simulink model "resolved_acceleration_control_final"  (R2016a)
settings: Solver=ode45  StartTime=0.0  StopTime=25  FixedStep=0.001  RelTol=1e-3
InitFcn:
  | clear all;
  | Kpx = 10;
  | Kix = 25;
  | Kpy = 10;
  | Kiy = 25;
  | Kvphi = 3;
  | Kpphi = 2.25;
  | 
  | Kem = 0.0059;
  | Kti = 0.0059;
  | Vd = 5.4;
  | R = 1.71;
  | r = 0.072;
  | eta = 0.83;
  | N = 19;
  | 
  | Jw = 8.1e-4
undefined symbols (not defined in the file or in its folder): alpha1, alpha2, alpha3, l1, l2, l3
libraries: simulink x1
settings Model: Creator=Pichau  LastModifiedBy=Pichau

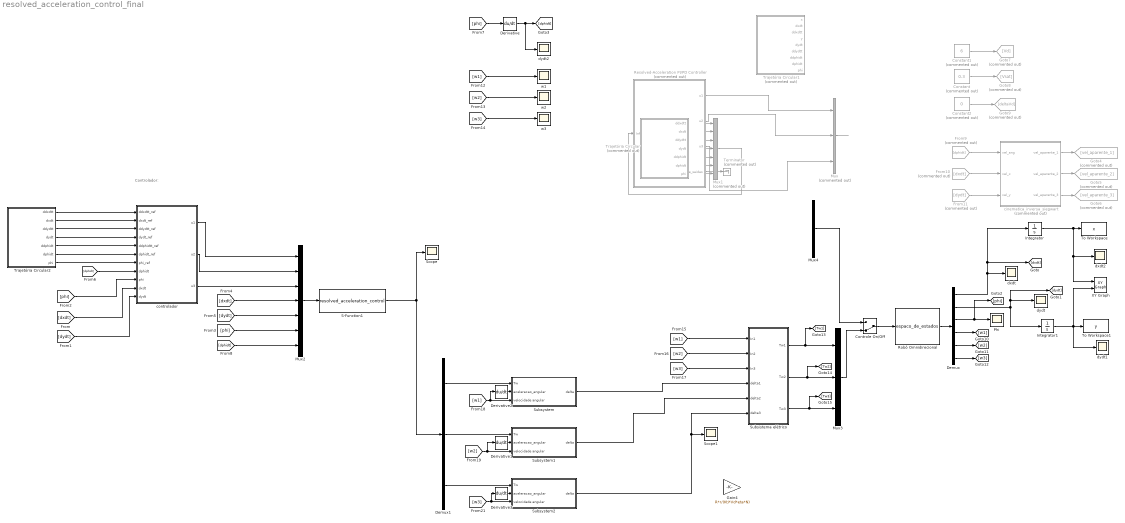
== system resolved_acceleration_control_final ==
  note: Controlador:
  Constant : Constant  Commented=on  Value=0.3
  Constant1 : Constant  Commented=on  Value=6
  Constant2 : Constant  Commented=on  Value=0
  Controle On/Off : ManualSwitch  CurrentSetting=0
  Demux : Demux  Outputs=6
  Demux1 : Demux  Outputs=3
  Derivative{,1..3} (4 alike) : Derivative
  From10 : From  Commented=on  GotoTag=dxdt
  From11 : From  Commented=on  GotoTag=dydt
  From9 : From  Commented=on  GotoTag=dphidt
  Gain4 : Gain  Gain=R*r/(Kti*Vd*eta*N)
  Goto4 : Goto  Commented=on  GotoTag=vel_aparente_1
  Goto5 : Goto  Commented=on  GotoTag=vel_aparente_2
  Goto6 : Goto  Commented=on  GotoTag=vel_aparente_3
  Goto7 : Goto  Commented=on  GotoTag=Vd
  Goto8 : Goto  Commented=on  GotoTag=Vsat
  Goto9 : Goto  Commented=on  GotoTag=deltaVd
  Integrator : Integrator  InitialCondition=0.3
  Integrator1 : Integrator
  Mux : Mux  Commented=on  Inputs=3
  Mux1 : Mux  Commented=on  Inputs=7
  Mux2 : Mux  Inputs=7
  Mux3 : Mux  Inputs=3
  Mux4 : Mux  Inputs=3
  Phi : Scope
  Resolved-Acceleration PI/PD Controller : Subsystem  Commented=on  mask{m=9.4, r=0.0245, L=11.25, J=11.25, Jw=0.02108, Kpx=10, Kix=25, Kpy=10, Kiy=25, Kvphi=3, Kpphi=2.25}
  Robô Omnidirecional : S-Function  FunctionName=espaco_de_estados  Parameters=r,m,Jw,J,L  SFunctionDeploymentMode=off  EnableBusSupport=off  mask{r=0.072, m=1.71, Jw=8.1e-4, J=2.125, L=0.09}
      mask prompts: r "r (m)"; m "m (Kg)"; Jw "Jw (Kg*m^2)"; J "J (Kg*m^2)"; L "L (m)"
      mask Display: image(imread('Robot_omnidirectional_drive.png'));
  S-Function1 : S-Function  FunctionName=resolved_acceleration_control  Parameters=r,L,m,J,Jw  SFunctionDeploymentMode=off  EnableBusSupport=off  mask{r=0.072, L=0.09, m=1.71, J=2.125, Jw=8.1e-4}
  Scope : Scope
  Scope1 : Scope
  Subsistema elétrico : Subsystem
  Subsystem : Subsystem
  Subsystem1 : Subsystem
  Subsystem2 : Subsystem
  Terminator : Terminator  Commented=on
  To Workspace : ToWorkspace  VariableName=x  SaveFormat=Timeseries  SampleTime=-1
  To Workspace1 : ToWorkspace  VariableName=y  SaveFormat=Timeseries  SampleTime=-1
  Trajetória Circular : Subsystem  Commented=on
  Trajetória Circular1 : Subsystem  Commented=on
  Trajetória Circular2 : Subsystem
  XY Graph : simulink/Sinks/XY Graph  xmin=-1  xmax=1  ymin=-1  ymax=1  st=-1
  cinematica_inversa_siegwart : Subsystem  Commented=on
  controlador : Subsystem
  dxdt : Scope
  dxdt2 : Scope
  dydt : Scope
  dydt1 : Scope
  dydt2 : Scope
  w1 : Scope
  w2 : Scope
  w3 : Scope
  wires:
  Mux/1 -> ?
  Robô Omnidirecional/1 -> Demux/1
  Resolved-Acceleration PI/PD Controller/4(vetor_de_saidas) -> Terminator/1
  Trajetória Circular/1(ddxdtt) -> Mux1/1
  Trajetória Circular/2(dxdt) -> Mux1/2
  Trajetória Circular/3(ddydtt) -> Mux1/3
  Trajetória Circular/4(dydt) -> Mux1/4
  Trajetória Circular/5(ddphidt) -> Mux1/5
  Trajetória Circular/6(dphidt) -> Mux1/6
  Trajetória Circular/7(phi) -> Mux1/7
  Mux1/1 -> Resolved-Acceleration PI/PD Controller/1(Informação da trajetória)
  Integrator1/1 -> XY Graph/2, To Workspace1/1, dydt1/1
  Integrator/1 -> XY Graph/1, dxdt2/1, To Workspace/1
  Trajetória Circular2/2(dxdt) -> controlador/2(dxdt_ref)
  Trajetória Circular2/6(dphidt) -> controlador/6(dphidt_ref)
  Trajetória Circular2/1(ddxdtt) -> controlador/1(ddxdtt_ref)
  Trajetória Circular2/4(dydt) -> controlador/4(dydt_ref)
  Trajetória Circular2/3(ddydtt) -> controlador/3(ddydtt_ref)
  Trajetória Circular2/7(phi) -> controlador/7(phi_ref)
  Trajetória Circular2/5(ddphidt) -> controlador/5(ddphidtt_ref)
  controlador/1(u1) -> Mux2/1
  controlador/2(u2) -> Mux2/2
  controlador/3(u3) -> Mux2/3
  [dxdt] -> controlador/10(dxdt)
  [dydt] -> controlador/11(dydt)
  [phi] -> controlador/9(phi)
  Resolved-Acceleration PI/PD Controller/1(u1) -> Mux/1
  Resolved-Acceleration PI/PD Controller/2(u2) -> Mux/2
  Resolved-Acceleration PI/PD Controller/3(u3) -> Mux/3
  Mux2/1 -> S-Function1/1
  [dphidt] -> controlador/8(dphidt)
  Derivative/1 -> dydt2/1, [dphidt]
  S-Function1/1 -> Scope/1, Demux1/1
  Mux3/1 -> Controle On/Off/2
  Controle On/Off/1 -> Robô Omnidirecional/1
  From9/1 -> cinematica_inversa_siegwart/1(vel_ang)
  From10/1 -> cinematica_inversa_siegwart/2(vel_x)
  From11/1 -> cinematica_inversa_siegwart/3(vel_y)
  cinematica_inversa_siegwart/1(vel_aparente_1) -> Goto4/1
  cinematica_inversa_siegwart/2(vel_aparente_2) -> Goto5/1
  cinematica_inversa_siegwart/3(vel_aparente_3) -> Goto6/1
  Constant1/1 -> Goto7/1
  Constant/1 -> Goto8/1
  Constant2/1 -> Goto9/1
  [w3] -> w3/1
  [w2] -> w2/1
  [w1] -> w1/1
  Demux/1 -> [dxdt], Integrator/1, dxdt/1
  Demux/2 -> Integrator1/1, [dydt], dydt/1
  Demux/3 -> Phi/1, [phi]
  [phi] -> Derivative/1
  [dxdt] -> Mux2/4
  [dydt] -> Mux2/5
  [phi] -> Mux2/6
  [dphidt] -> Mux2/7
  Demux/4 -> [w1]
  Demux/5 -> [w2]
  Demux/6 -> [w3]
  [w1] -> Subsistema elétrico/1(In1)
  [w2] -> Subsistema elétrico/2(In2)
  [w3] -> Subsistema elétrico/3(In3)
  Subsistema elétrico/3(Tw3) -> [Tw3], Mux3/3
  Subsistema elétrico/2(Tw2) -> [Tw2], Mux3/2
  Subsistema elétrico/1(Tw1) -> [Tw1], Mux3/1
  Mux4/1 -> Controle On/Off/1
  Demux1/1 -> Subsystem/1(Tw)
  Demux1/2 -> Subsystem1/1(Tw)
  Demux1/3 -> Subsystem2/1(Tw)
  Subsystem1/1(delta) -> Subsistema elétrico/5(delta2)
  Subsystem2/1(delta) -> Subsistema elétrico/6(delta3), Scope1/1
  Subsystem/1(delta) -> Subsistema elétrico/4(delta1)
  [w1] -> Derivative2/1, Subsystem/3(velocidade angular)
  [w2] -> Derivative1/1, Subsystem1/3(velocidade angular)
  [w3] -> Derivative3/1, Subsystem2/3(velocidade angular)
  Derivative1/1 -> Subsystem1/2(aceleracao_angular)
  Derivative2/1 -> Subsystem/2(aceleracao_angular)
  Derivative3/1 -> Subsystem2/2(aceleracao_angular)

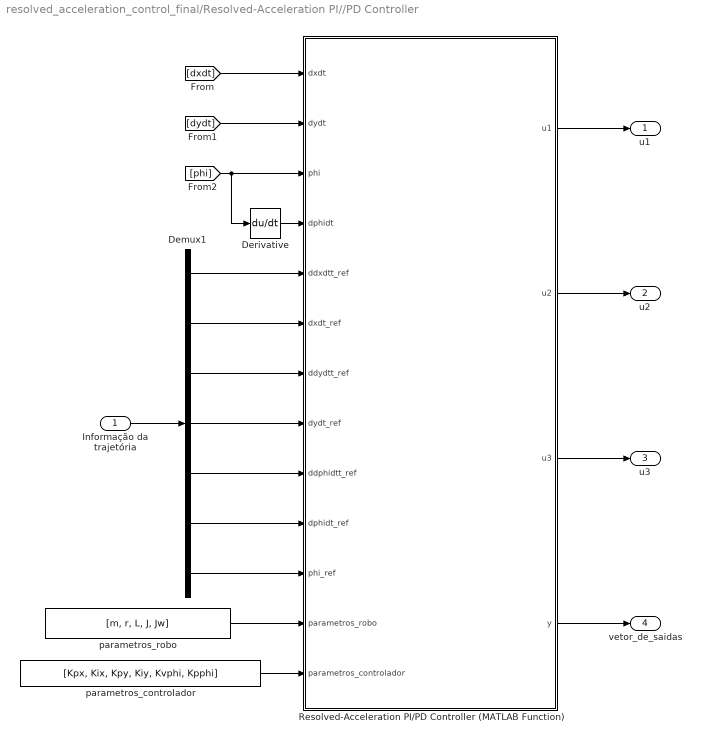
== system resolved_acceleration_control_final/Resolved-Acceleration PI//PD Controller ==
  Informação da trajetória : Inport
  Demux1 : Demux  Outputs=7
  Derivative : Derivative
  Resolved-Acceleration PI/PD Controller (MATLAB Function) : MATLAB Function  TreatAsAtomicUnit=on
  parametros_controlador : Constant  Value=[Kpx, Kix, Kpy, Kiy, Kvphi, Kpphi]
  parametros_robo : Constant  Value=[m, r, L, J, Jw]
  u1 : Outport
  u2 : Outport  Port=2
  u3 : Outport  Port=3
  vetor_de_saidas : Outport  Port=4
  wires:
  Resolved-Acceleration PI/PD Controller (MATLAB Function)/1(u1) -> u1/1
  parametros_controlador/1 -> Resolved-Acceleration PI/PD Controller (MATLAB Function)/13(parametros_controlador)
  [dxdt] -> Resolved-Acceleration PI/PD Controller (MATLAB Function)/1(dxdt)
  [phi] -> Derivative/1, Resolved-Acceleration PI/PD Controller (MATLAB Function)/3(phi)
  Resolved-Acceleration PI/PD Controller (MATLAB Function)/2(u2) -> u2/1
  Demux1/3 -> Resolved-Acceleration PI/PD Controller (MATLAB Function)/7(ddydtt_ref)
  Informação da trajetória/1 -> Demux1/1
  Resolved-Acceleration PI/PD Controller (MATLAB Function)/4(y) -> vetor_de_saidas/1
  parametros_robo/1 -> Resolved-Acceleration PI/PD Controller (MATLAB Function)/12(parametros_robo)
  Demux1/1 -> Resolved-Acceleration PI/PD Controller (MATLAB Function)/5(ddxdtt_ref)
  Demux1/2 -> Resolved-Acceleration PI/PD Controller (MATLAB Function)/6(dxdt_ref)
  Demux1/4 -> Resolved-Acceleration PI/PD Controller (MATLAB Function)/8(dydt_ref)
  Demux1/6 -> Resolved-Acceleration PI/PD Controller (MATLAB Function)/10(dphidt_ref)
  Derivative/1 -> Resolved-Acceleration PI/PD Controller (MATLAB Function)/4(dphidt)
  Resolved-Acceleration PI/PD Controller (MATLAB Function)/3(u3) -> u3/1
  Demux1/5 -> Resolved-Acceleration PI/PD Controller (MATLAB Function)/9(ddphidtt_ref)
  Demux1/7 -> Resolved-Acceleration PI/PD Controller (MATLAB Function)/11(phi_ref)
  [dydt] -> Resolved-Acceleration PI/PD Controller (MATLAB Function)/2(dydt)

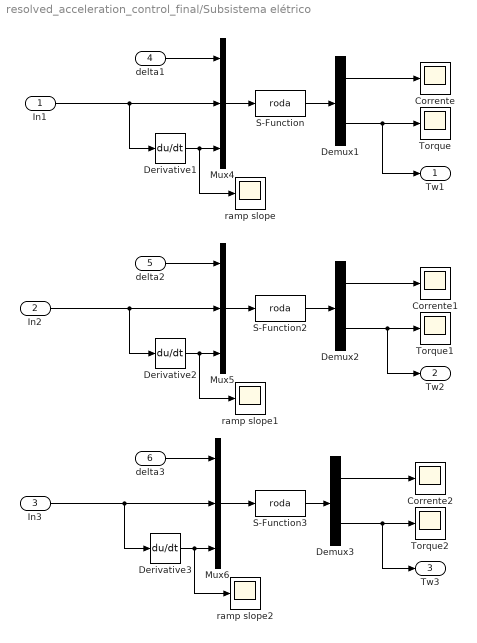
== system resolved_acceleration_control_final/Subsistema elétrico ==
  In1 : Inport
  In2 : Inport  Port=2
  In3 : Inport  Port=3
  delta1 : Inport  Port=4
  delta2 : Inport  Port=5
  delta3 : Inport  Port=6
  Corrente : Scope
  Corrente1 : Scope
  Corrente2 : Scope
  Demux1 : Demux  Outputs=2
  Demux2 : Demux  Outputs=2
  Demux3 : Demux  Outputs=2
  Derivative1 : Derivative
  Derivative2 : Derivative
  Derivative3 : Derivative
  Mux4 : Mux  Inputs=3
  Mux5 : Mux  Inputs=3
  Mux6 : Mux  Inputs=3
  S-Function : S-Function  FunctionName=roda  Parameters=Vd,Vsat,deltaVd,L,Kem,R,Kti,Jm,eta,N  SFunctionDeploymentMode=off  EnableBusSupport=off  mask{Vd=6, Vsat=0.3, deltaVd=0, L=0.00011, Kem=0.0059, R=1.71, Kti=0.0059, Jm=3.88e-7, eta=0.83, N=19}
  S-Function2 : S-Function  FunctionName=roda  Parameters=Vd,Vsat,deltaVd,L,Kem,R,Kti,Jm,eta,N  SFunctionDeploymentMode=off  EnableBusSupport=off  mask{Vd=6, Vsat=0.3, deltaVd=0, L=0.00011, Kem=0.0059, R=1.71, Kti=0.0059, Jm=3.88e-7, eta=0.83, N=19}
  S-Function3 : S-Function  FunctionName=roda  Parameters=Vd,Vsat,deltaVd,L,Kem,R,Kti,Jm,eta,N  SFunctionDeploymentMode=off  EnableBusSupport=off  mask{Vd=6, Vsat=0.3, deltaVd=0, L=0.00011, Kem=0.0059, R=1.71, Kti=0.0059, Jm=3.88e-7, eta=0.83, N=19}
  Torque : Scope
  Torque1 : Scope
  Torque2 : Scope
  ramp slope : Scope
  ramp slope1 : Scope
  ramp slope2 : Scope
  Tw1 : Outport
  Tw2 : Outport  Port=2
  Tw3 : Outport  Port=3
  wires:
  Demux3/1 -> Corrente2/1
  Mux6/1 -> S-Function3/1
  Derivative3/1 -> ramp slope2/1, Mux6/3
  Demux3/2 -> Tw3/1, Torque2/1
  In3/1 -> Mux6/2, Derivative3/1
  S-Function3/1 -> Demux3/1
  delta2/1 -> Mux5/1
  delta3/1 -> Mux6/1
  Mux5/1 -> S-Function2/1
  In2/1 -> Derivative2/1, Mux5/2
  S-Function2/1 -> Demux2/1
  Demux2/1 -> Corrente1/1
  Demux2/2 -> Tw2/1, Torque1/1
  Derivative2/1 -> Mux5/3, ramp slope1/1
  Derivative1/1 -> ramp slope/1, Mux4/3
  In1/1 -> Mux4/2, Derivative1/1
  Demux1/2 -> Tw1/1, Torque/1
  Mux4/1 -> S-Function/1
  S-Function/1 -> Demux1/1
  delta1/1 -> Mux4/1
  Demux1/1 -> Corrente/1

== system resolved_acceleration_control_final/Subsystem ==
  Tw : Inport
  aceleracao_angular : Inport  Port=2
  velocidade angular : Inport  Port=3
  Add : Sum  Inputs=+++
  Gain : Gain  Gain=R/(eta*N*Kti*Vd)
  Gain1 : Gain  Gain=Kem
  Gain2 : Gain  Gain=R*Jw/(eta*N^2*Kti*Vd)
  delta : Outport
  wires:
  aceleracao_angular/1 -> Gain2/1
  velocidade angular/1 -> Gain1/1
  Add/1 -> delta/1
  Tw/1 -> Gain/1
  Gain1/1 -> Add/3
  Gain/1 -> Add/1
  Gain2/1 -> Add/2

== system resolved_acceleration_control_final/Subsystem1 ==
  Tw : Inport
  aceleracao_angular : Inport  Port=2
  velocidade angular : Inport  Port=3
  Add : Sum  Inputs=+++
  Gain : Gain  Gain=R/(eta*N*Kti*Vd)
  Gain1 : Gain  Gain=Kem
  Gain2 : Gain  Gain=R*Jw/(eta*N^2*Kti*Vd)
  delta : Outport
  wires:
  Gain2/1 -> Add/2
  Gain/1 -> Add/1
  Gain1/1 -> Add/3
  Tw/1 -> Gain/1
  Add/1 -> delta/1
  velocidade angular/1 -> Gain1/1
  aceleracao_angular/1 -> Gain2/1

== system resolved_acceleration_control_final/Subsystem2 ==
  Tw : Inport
  aceleracao_angular : Inport  Port=2
  velocidade angular : Inport  Port=3
  Add : Sum  Inputs=+++
  Gain : Gain  Gain=R/(eta*N*Kti*Vd)
  Gain1 : Gain  Gain=Kem
  Gain2 : Gain  Gain=R*Jw/(eta*N^2*Kti*Vd)
  delta : Outport
  wires:
  aceleracao_angular/1 -> Gain2/1
  velocidade angular/1 -> Gain1/1
  Add/1 -> delta/1
  Tw/1 -> Gain/1
  Gain1/1 -> Add/3
  Gain/1 -> Add/1
  Gain2/1 -> Add/2

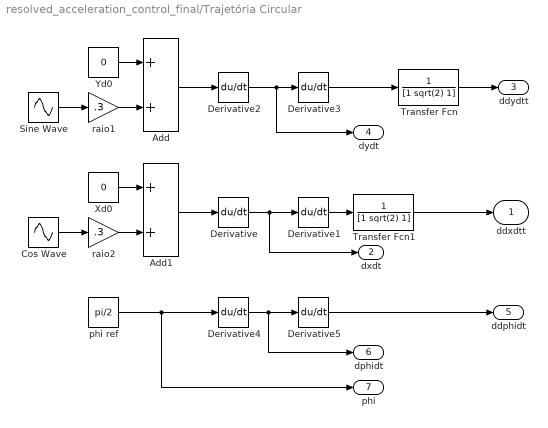
== system resolved_acceleration_control_final/Trajetória Circular ==
  Add : Sum
  Add1 : Sum
  Cos Wave : Sin  Frequency=0.3  Phase=pi/2  SampleTime=0
  Derivative{,1..5} (6 alike) : Derivative
  Sine Wave : Sin  Frequency=0.3  SampleTime=0
  Transfer Fcn : TransferFcn  Denominator=[1 sqrt(2) 1]
  Transfer Fcn1 : TransferFcn  Denominator=[1 sqrt(2) 1]
  Xd0 : Constant  Value=0
  Yd0 : Constant  Value=0
  phi ref : Constant  Value=pi/2
  raio1 : Gain  Gain=.3
  raio2 : Gain  Gain=.3
  ddxdtt : Outport
  dxdt : Outport  Port=2
  ddydtt : Outport  Port=3
  dydt : Outport  Port=4
  ddphidt : Outport  Port=5
  dphidt : Outport  Port=6
  phi : Outport  Port=7
  wires:
  Yd0/1 -> Add/1
  Xd0/1 -> Add1/1
  Cos Wave/1 -> raio2/1
  raio2/1 -> Add1/2
  Add1/1 -> Derivative/1
  Add/1 -> Derivative2/1
  raio1/1 -> Add/2
  Sine Wave/1 -> raio1/1
  Derivative/1 -> dxdt/1, Derivative1/1
  Derivative2/1 -> dydt/1, Derivative3/1
  Derivative3/1 -> Transfer Fcn/1
  Derivative1/1 -> Transfer Fcn1/1
  Derivative4/1 -> dphidt/1, Derivative5/1
  Derivative5/1 -> ddphidt/1
  phi ref/1 -> phi/1, Derivative4/1
  Transfer Fcn/1 -> ddydtt/1
  Transfer Fcn1/1 -> ddxdtt/1

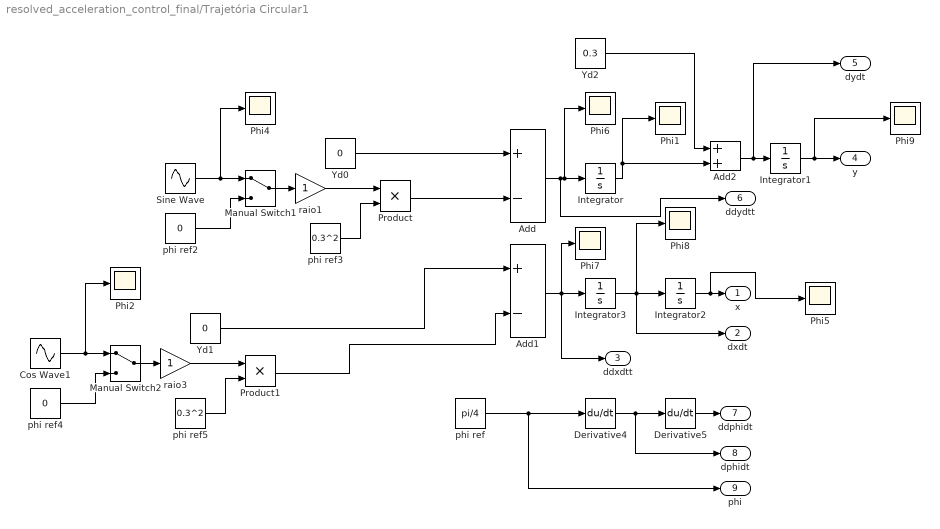
== system resolved_acceleration_control_final/Trajetória Circular1 ==
  Add : Sum  Inputs=+-
  Add1 : Sum  Inputs=+-
  Add2 : Sum
  Cos Wave1 : Sin  Frequency=0.3  Phase=pi/2  SampleTime=0
  Derivative4 : Derivative
  Derivative5 : Derivative
  Integrator : Integrator
  Integrator1 : Integrator
  Integrator2 : Integrator  InitialCondition=1
  Integrator3 : Integrator
  Manual Switch1 : ManualSwitch
  Manual Switch2 : ManualSwitch
  Phi{1..2,4..9} (8 alike) : Scope
  Product : Product
  Product1 : Product
  Sine Wave : Sin  Frequency=0.3  SampleTime=0
  Yd0 : Constant  Value=0
  Yd1 : Constant  Value=0
  Yd2 : Constant  Value=0.3
  phi ref : Constant  Value=pi/4
  phi ref2 : Constant  Value=0
  phi ref3 : Constant  Value=0.3^2
  phi ref4 : Constant  Value=0
  phi ref5 : Constant  Value=0.3^2
  raio1 : Gain
  raio3 : Gain
  x : Outport
  dxdt : Outport  Port=2
  ddxdtt : Outport  Port=3
  y : Outport  Port=4
  dydt : Outport  Port=5
  ddydtt : Outport  Port=6
  ddphidt : Outport  Port=7
  dphidt : Outport  Port=8
  phi : Outport  Port=9
  wires:
  phi ref/1 -> Derivative4/1, phi/1
  Derivative5/1 -> ddphidt/1
  Derivative4/1 -> Derivative5/1, dphidt/1
  Integrator/1 -> Phi1/1, Add2/2
  Integrator3/1 -> Phi8/1, Integrator2/1, dxdt/1
  Sine Wave/1 -> Phi4/1, Manual Switch1/1
  raio1/1 -> Product/1
  Add1/1 -> ddxdtt/1, Phi7/1, Integrator3/1
  Product1/1 -> Add1/2
  Yd1/1 -> Add1/1
  Yd0/1 -> Add/1
  Manual Switch1/1 -> raio1/1
  phi ref2/1 -> Manual Switch1/2
  Product/1 -> Add/2
  phi ref3/1 -> Product/2
  Cos Wave1/1 -> Phi2/1, Manual Switch2/1
  raio3/1 -> Product1/1
  Manual Switch2/1 -> raio3/1
  phi ref4/1 -> Manual Switch2/2
  phi ref5/1 -> Product1/2
  Integrator1/1 -> Phi9/1, y/1
  Integrator2/1 -> Phi5/1, x/1
  Add/1 -> ddydtt/1, Phi6/1, Integrator/1
  Yd2/1 -> Add2/1
  Add2/1 -> dydt/1, Integrator1/1

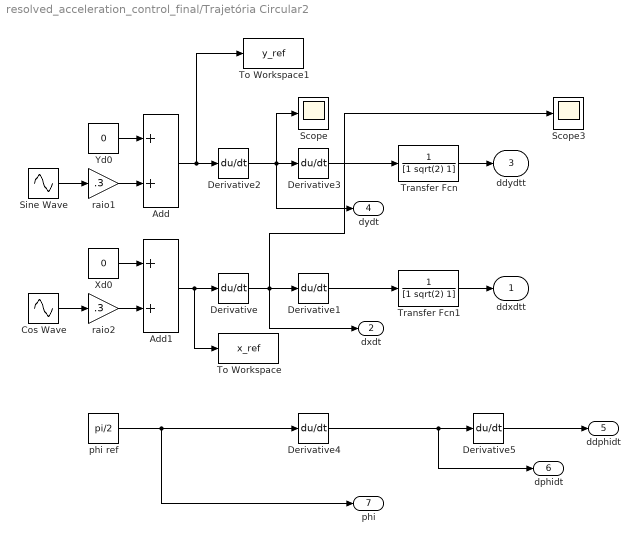
== system resolved_acceleration_control_final/Trajetória Circular2 ==
  Add : Sum
  Add1 : Sum
  Cos Wave : Sin  Frequency=0.3  Phase=pi/2  SampleTime=0
  Derivative{,1..5} (6 alike) : Derivative
  Scope : Scope
  Scope3 : Scope
  Sine Wave : Sin  Frequency=0.3  SampleTime=0
  To Workspace : ToWorkspace  VariableName=x_ref  SaveFormat=Timeseries  SampleTime=-1
  To Workspace1 : ToWorkspace  VariableName=y_ref  SaveFormat=Timeseries  SampleTime=-1
  Transfer Fcn : TransferFcn  Denominator=[1 sqrt(2) 1]
  Transfer Fcn1 : TransferFcn  Denominator=[1 sqrt(2) 1]
  Xd0 : Constant  Value=0
  Yd0 : Constant  Value=0
  phi ref : Constant  Value=pi/2
  raio1 : Gain  Gain=.3
  raio2 : Gain  Gain=.3
  ddxdtt : Outport
  dxdt : Outport  Port=2
  ddydtt : Outport  Port=3
  dydt : Outport  Port=4
  ddphidt : Outport  Port=5
  dphidt : Outport  Port=6
  phi : Outport  Port=7
  wires:
  Transfer Fcn1/1 -> ddxdtt/1
  Transfer Fcn/1 -> ddydtt/1
  Derivative5/1 -> ddphidt/1
  Derivative1/1 -> Transfer Fcn1/1
  Derivative3/1 -> Transfer Fcn/1
  Derivative2/1 -> Derivative3/1, Scope/1, dydt/1
  Derivative/1 -> Scope3/1, Derivative1/1, dxdt/1
  Sine Wave/1 -> raio1/1
  raio1/1 -> Add/2
  Add/1 -> To Workspace1/1, Derivative2/1
  Add1/1 -> To Workspace/1, Derivative/1
  raio2/1 -> Add1/2
  Cos Wave/1 -> raio2/1
  Xd0/1 -> Add1/1
  Yd0/1 -> Add/1
  phi ref/1 -> Derivative4/1, phi/1
  Derivative4/1 -> Derivative5/1, dphidt/1

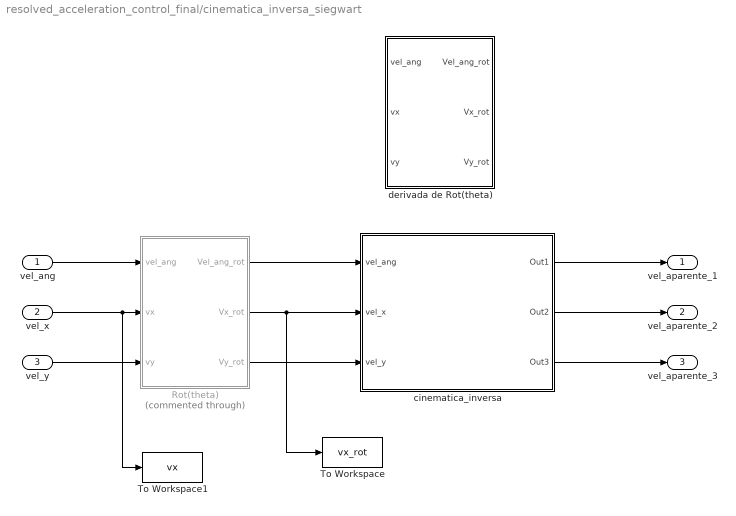
== system resolved_acceleration_control_final/cinematica_inversa_siegwart ==
  vel_ang : Inport
  vel_x : Inport  Port=2
  vel_y : Inport  Port=3
  Rot(theta) : Subsystem  Commented=through
  To Workspace : ToWorkspace  VariableName=vx_rot  SampleTime=-1
      settings: Save2DSignal=2-D array (concatenate along first dimension)
  To Workspace1 : ToWorkspace  VariableName=vx  SampleTime=-1
      settings: Save2DSignal=2-D array (concatenate along first dimension)
  cinematica_inversa : Subsystem
  derivada de Rot(theta) : Subsystem
  vel_aparente_1 : Outport
  vel_aparente_2 : Outport  Port=2
  vel_aparente_3 : Outport  Port=3
  wires:
  vel_ang/1 -> Rot(theta)/1(vel_ang)
  vel_x/1 -> To Workspace1/1, Rot(theta)/2(vx)
  vel_y/1 -> Rot(theta)/3(vy)
  Rot(theta)/2(Vx_rot) -> To Workspace/1, cinematica_inversa/2(vel_x)
  Rot(theta)/3(Vy_rot) -> cinematica_inversa/3(vel_y)
  Rot(theta)/1(Vel_ang_rot) -> cinematica_inversa/1(vel_ang)
  cinematica_inversa/1(Out1) -> vel_aparente_1/1
  cinematica_inversa/2(Out2) -> vel_aparente_2/1
  cinematica_inversa/3(Out3) -> vel_aparente_3/1

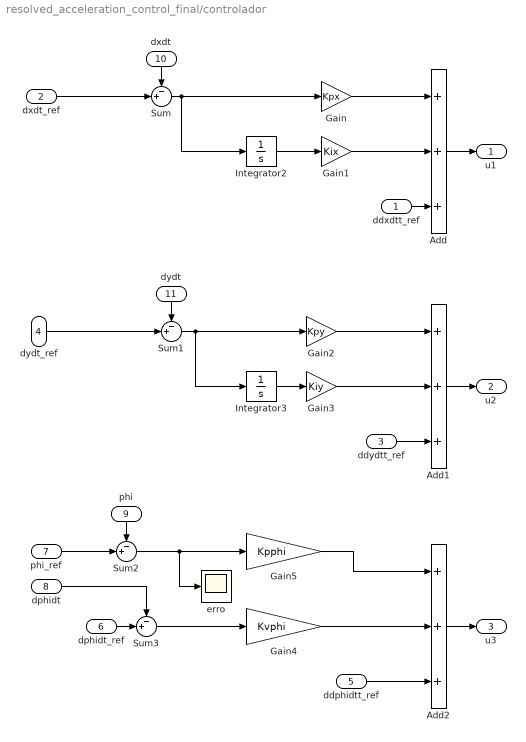
== system resolved_acceleration_control_final/controlador ==
  ddxdtt_ref : Inport
  dxdt_ref : Inport  Port=2
  ddydtt_ref : Inport  Port=3
  dydt_ref : Inport  Port=4
  ddphidtt_ref : Inport  Port=5
  dphidt_ref : Inport  Port=6
  phi_ref : Inport  Port=7
  dphidt : Inport  Port=8
  phi : Inport  Port=9
  dxdt : Inport  Port=10
  dydt : Inport  Port=11
  Add : Sum  Inputs=+++
  Add1 : Sum  Inputs=+++
  Add2 : Sum  Inputs=+++
  Gain : Gain  Gain=Kpx
  Gain1 : Gain  Gain=Kix
  Gain2 : Gain  Gain=Kpy
  Gain3 : Gain  Gain=Kiy
  Gain4 : Gain  Gain=Kvphi
  Gain5 : Gain  Gain=Kpphi
  Integrator2 : Integrator
  Integrator3 : Integrator
  Sum{,1..3} (4 alike) : Sum  Inputs=-+|
  erro : Scope
  u1 : Outport
  u2 : Outport  Port=2
  u3 : Outport  Port=3
  wires:
  Sum2/1 -> Gain5/1, erro/1
  Sum1/1 -> Gain2/1, Integrator3/1
  Gain1/1 -> Add/2
  Integrator2/1 -> Gain1/1
  dydt_ref/1 -> Sum1/2
  Add/1 -> u1/1
  Gain2/1 -> Add1/1
  Integrator3/1 -> Gain3/1
  dphidt/1 -> Sum3/1
  Gain4/1 -> Add2/2
  Sum/1 -> Gain/1, Integrator2/1
  Gain3/1 -> Add1/2
  Gain5/1 -> Add2/1
  Sum3/1 -> Gain4/1
  ddphidtt_ref/1 -> Add2/3
  ddydtt_ref/1 -> Add1/3
  Add1/1 -> u2/1
  ddxdtt_ref/1 -> Add/3
  phi/1 -> Sum2/1
  Add2/1 -> u3/1
  dxdt_ref/1 -> Sum/2
  dxdt/1 -> Sum/1
  phi_ref/1 -> Sum2/2
  Gain/1 -> Add/1
  dydt/1 -> Sum1/1
  dphidt_ref/1 -> Sum3/2

== system resolved_acceleration_control_final/cinematica_inversa_siegwart/Rot(theta) ==
  vel_ang : Inport
  vx : Inport  Port=2
  vy : Inport  Port=3
  Integrator : Integrator
  Subsystem3 : Subsystem
  Subsystem4 : Subsystem
  Vel_ang_rot : Outport
  Vx_rot : Outport  Port=2
  Vy_rot : Outport  Port=3
  wires:
  Subsystem3/1(vx_rot) -> Vx_rot/1
  Subsystem4/1(vy_rot) -> Vy_rot/1
  vx/1 -> Subsystem4/2(vx), Subsystem3/2(vx)
  vy/1 -> Subsystem4/3(vy), Subsystem3/3(vy)
  vel_ang/1 -> Vel_ang_rot/1, Integrator/1
  Integrator/1 -> Subsystem4/1(theta), Subsystem3/1(theta)

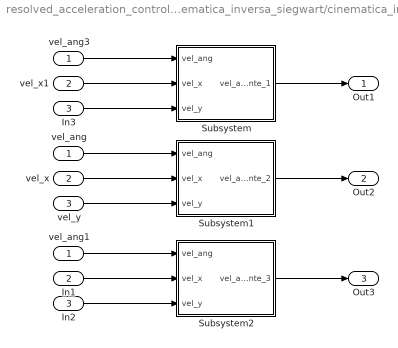
== system resolved_acceleration_control_final/cinematica_inversa_siegwart/cinematica_inversa ==
  vel_ang : Inport
  vel_x : Inport  Port=2
  vel_y : Inport  Port=3
  In1 : InportShadow  Port=2
  In2 : InportShadow  Port=3
  In3 : InportShadow  Port=3
  Subsystem : Subsystem
  Subsystem1 : Subsystem
  Subsystem2 : Subsystem
  vel_ang1 : InportShadow
  vel_ang3 : InportShadow
  vel_x1 : InportShadow  Port=2
  Out1 : Outport
  Out2 : Outport  Port=2
  Out3 : Outport  Port=3
  wires:
  Subsystem/1(vel_aparente_1) -> Out1/1
  vel_x/1 -> Subsystem1/2(vel_x)
  vel_ang/1 -> Subsystem1/1(vel_ang)
  vel_y/1 -> Subsystem1/3(vel_y)
  Subsystem1/1(vel_aparente_2) -> Out2/1
  Subsystem2/1(vel_aparente_3) -> Out3/1
  vel_ang3/1 -> Subsystem/1(vel_ang)
  vel_x1/1 -> Subsystem/2(vel_x)
  vel_ang1/1 -> Subsystem2/1(vel_ang)
  In1/1 -> Subsystem2/2(vel_x)
  In2/1 -> Subsystem2/3(vel_y)
  In3/1 -> Subsystem/3(vel_y)

== system resolved_acceleration_control_final/cinematica_inversa_siegwart/derivada de Rot(theta) ==
  vel_ang : Inport
  vx : Inport  Port=2
  vy : Inport  Port=3
  Integrator : Integrator
  Subsystem3 : Subsystem
  Subsystem4 : Subsystem
  Vel_ang_rot : Outport
  Vx_rot : Outport  Port=2
  Vy_rot : Outport  Port=3
  wires:
  Subsystem3/1(vx_rot) -> Vx_rot/1
  Subsystem4/1(vy_rot) -> Vy_rot/1
  vx/1 -> Subsystem4/2(vx), Subsystem3/2(vx)
  vy/1 -> Subsystem4/3(vy), Subsystem3/3(vy)
  vel_ang/1 -> Vel_ang_rot/1, Integrator/1
  Integrator/1 -> Subsystem4/1(theta), Subsystem3/1(theta)

== system resolved_acceleration_control_final/cinematica_inversa_siegwart/Rot(theta)/Subsystem3 ==
  theta : Inport
  vx : Inport  Port=2
  vy : Inport  Port=3
  Add : Sum
  Divide : Product  Inputs=**
  Divide1 : Product  Inputs=**
  Trigonometric Function : Trigonometry
  Trigonometric Function1 : Trigonometry  Operator=cos
  vx_rot : Outport
  wires:
  Divide/1 -> Add/1
  Trigonometric Function/1 -> Divide1/1
  theta/1 -> Trigonometric Function1/1, Trigonometric Function/1
  Add/1 -> vx_rot/1
  Divide1/1 -> Add/2
  Trigonometric Function1/1 -> Divide/1
  vy/1 -> Divide1/2
  vx/1 -> Divide/2

== system resolved_acceleration_control_final/cinematica_inversa_siegwart/Rot(theta)/Subsystem4 ==
  theta : Inport
  vx : Inport  Port=2
  vy : Inport  Port=3
  Add : Sum  Inputs=-+
  Divide : Product  Inputs=**
  Divide1 : Product  Inputs=**
  Trigonometric Function : Trigonometry  Operator=cos
  Trigonometric Function1 : Trigonometry
  vy_rot : Outport
  wires:
  vx/1 -> Divide/2
  vy/1 -> Divide1/2
  Trigonometric Function1/1 -> Divide/1
  Divide1/1 -> Add/2
  Add/1 -> vy_rot/1
  theta/1 -> Trigonometric Function/1, Trigonometric Function1/1
  Trigonometric Function/1 -> Divide1/1
  Divide/1 -> Add/1

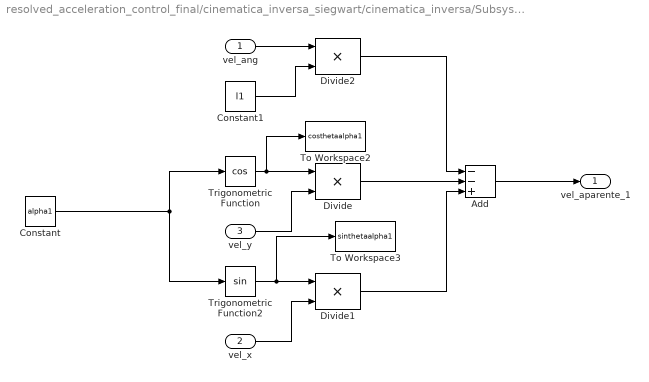
== system resolved_acceleration_control_final/cinematica_inversa_siegwart/cinematica_inversa/Subsystem ==
  vel_ang : Inport
  vel_x : Inport  Port=2
  vel_y : Inport  Port=3
  Add : Sum  Inputs=--+
  Constant : Constant  Value=alpha1
  Constant1 : Constant  Value=l1
  Divide : Product  Inputs=**
  Divide1 : Product  Inputs=**
  Divide2 : Product  Inputs=**
  To Workspace2 : ToWorkspace  VariableName=costhetaalpha1  SampleTime=-1
      settings: Save2DSignal=2-D array (concatenate along first dimension)
  To Workspace3 : ToWorkspace  VariableName=sinthetaalpha1  SampleTime=-1
      settings: Save2DSignal=2-D array (concatenate along first dimension)
  Trigonometric Function : Trigonometry  Operator=cos
  Trigonometric Function2 : Trigonometry
  vel_aparente_1 : Outport
  wires:
  vel_y/1 -> Divide/2
  vel_ang/1 -> Divide2/1
  Trigonometric Function/1 -> To Workspace2/1, Divide/1
  Constant/1 -> Trigonometric Function/1, Trigonometric Function2/1
  Trigonometric Function2/1 -> To Workspace3/1, Divide1/1
  vel_x/1 -> Divide1/2
  Divide/1 -> Add/2
  Divide1/1 -> Add/3
  Constant1/1 -> Divide2/2
  Divide2/1 -> Add/1
  Add/1 -> vel_aparente_1/1

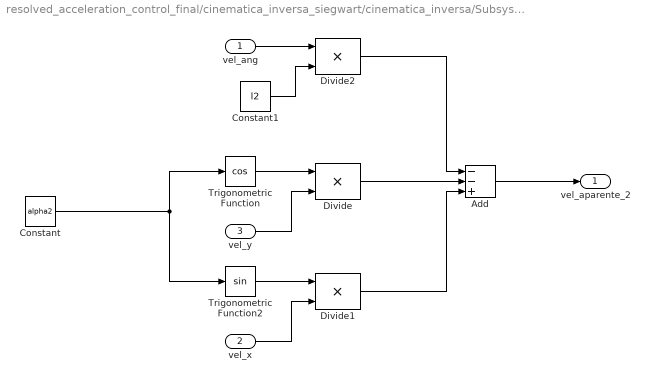
== system resolved_acceleration_control_final/cinematica_inversa_siegwart/cinematica_inversa/Subsystem1 ==
  vel_ang : Inport
  vel_x : Inport  Port=2
  vel_y : Inport  Port=3
  Add : Sum  Inputs=--+
  Constant : Constant  Value=alpha2
  Constant1 : Constant  Value=l2
  Divide : Product  Inputs=**
  Divide1 : Product  Inputs=**
  Divide2 : Product  Inputs=**
  Trigonometric Function : Trigonometry  Operator=cos
  Trigonometric Function2 : Trigonometry
  vel_aparente_2 : Outport
  wires:
  Add/1 -> vel_aparente_2/1
  Divide2/1 -> Add/1
  Constant1/1 -> Divide2/2
  Divide1/1 -> Add/3
  Divide/1 -> Add/2
  vel_x/1 -> Divide1/2
  Trigonometric Function2/1 -> Divide1/1
  Constant/1 -> Trigonometric Function2/1, Trigonometric Function/1
  Trigonometric Function/1 -> Divide/1
  vel_ang/1 -> Divide2/1
  vel_y/1 -> Divide/2

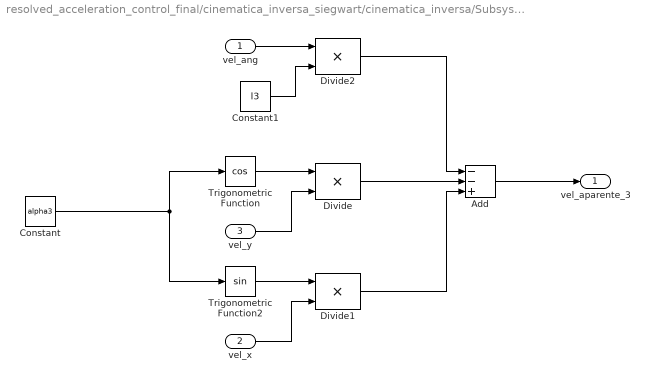
== system resolved_acceleration_control_final/cinematica_inversa_siegwart/cinematica_inversa/Subsystem2 ==
  vel_ang : Inport
  vel_x : Inport  Port=2
  vel_y : Inport  Port=3
  Add : Sum  Inputs=--+
  Constant : Constant  Value=alpha3
  Constant1 : Constant  Value=l3
  Divide : Product  Inputs=**
  Divide1 : Product  Inputs=**
  Divide2 : Product  Inputs=**
  Trigonometric Function : Trigonometry  Operator=cos
  Trigonometric Function2 : Trigonometry
  vel_aparente_3 : Outport
  wires:
  vel_y/1 -> Divide/2
  vel_ang/1 -> Divide2/1
  Trigonometric Function/1 -> Divide/1
  Constant/1 -> Trigonometric Function/1, Trigonometric Function2/1
  Trigonometric Function2/1 -> Divide1/1
  vel_x/1 -> Divide1/2
  Divide/1 -> Add/2
  Divide1/1 -> Add/3
  Constant1/1 -> Divide2/2
  Divide2/1 -> Add/1
  Add/1 -> vel_aparente_3/1

== system resolved_acceleration_control_final/cinematica_inversa_siegwart/derivada de Rot(theta)/Subsystem3 ==
  theta : Inport
  vx : Inport  Port=2
  vy : Inport  Port=3
  Add : Sum
  Divide : Product  Inputs=**
  Divide1 : Product  Inputs=**
  Trigonometric Function : Trigonometry
  Trigonometric Function1 : Trigonometry  Operator=cos
  vx_rot : Outport
  wires:
  Divide/1 -> Add/1
  Trigonometric Function/1 -> Divide1/1
  theta/1 -> Trigonometric Function1/1, Trigonometric Function/1
  Add/1 -> vx_rot/1
  Divide1/1 -> Add/2
  Trigonometric Function1/1 -> Divide/1
  vy/1 -> Divide1/2
  vx/1 -> Divide/2

== system resolved_acceleration_control_final/cinematica_inversa_siegwart/derivada de Rot(theta)/Subsystem4 ==
  theta : Inport
  vx : Inport  Port=2
  vy : Inport  Port=3
  Add : Sum  Inputs=-+
  Divide : Product  Inputs=**
  Divide1 : Product  Inputs=**
  Trigonometric Function : Trigonometry  Operator=cos
  Trigonometric Function1 : Trigonometry
  vy_rot : Outport
  wires:
  vx/1 -> Divide/2
  vy/1 -> Divide1/2
  Trigonometric Function1/1 -> Divide/1
  Divide1/1 -> Add/2
  Add/1 -> vy_rot/1
  theta/1 -> Trigonometric Function/1, Trigonometric Function1/1
  Trigonometric Function/1 -> Divide1/1
  Divide/1 -> Add/1

== matlab function resolved_acceleration_control_final/Resolved-Acceleration PI//PD Controller/Resolved-Acceleration PI//PD Controller (MATLAB Function) ==
  data: dxdt input; u1 output; dydt input; phi input; dphidt input; ddxdtt_ref input; dxdt_ref input; ddydtt_ref input; dydt_ref input; ddphidtt_ref input; dphidt_ref input; phi_ref input; u2 output; u3 output; y output; parametros_robo input; parametros_controlador input
function [u1,u2,u3,y]= fcn(dxdt, dydt, phi, dphidt, ddxdtt_ref, dxdt_ref, ddydtt_ref, dydt_ref, ddphidtt_ref, dphidt_ref, phi_ref, parametros_robo, parametros_controlador)
%% Parâmetros do robô
m = parametros_robo(1);
r = parametros_robo(2);
L = parametros_robo(3);
J = parametros_robo(4);
Jw = parametros_robo(5);

%% Parâmetros do controlador
Kpx = parametros_controlador(1);
Kix = parametros_controlador(2);
Kpy = parametros_controlador(3);
Kiy = parametros_controlador(4);
Kvphi = parametros_controlador(5);
Kpphi = parametros_controlador(6);
%%
a2 = 3*Jw/(2*r^2*m+3*Jw);
b1 = r/(2*r^2*m+3*Jw);
b2 = r*L/(J*r^2+3*Jw*L^2);
beta1 = sin(phi)-sqrt(3)*cos(phi);
beta2 = sin(phi)+sqrt(3)*cos(phi);
beta3 = sqrt(3)*sin(phi)+cos(phi);
beta4 = cos(phi)-sqrt(3)*sin(phi);

persistent integral_of_x_error;
persistent integral_of_y_error;

xError = dxdt_ref-dxdt;
yError = dydt_ref-dydt;

if isempty(integral_of_x_error)
    integral_of_x_error = xError;   
else
    integral_of_x_error = integral_of_x_error+xError;
end

if isempty(integral_of_y_error)
    integral_of_y_error = yError;
else
    integral_of_y_error = integral_of_y_error+yError;
end

ddxodtt = ddxdtt_ref+Kpx*(dxdt_ref-dxdt)+Kix*integral_of_x_error;
ddyodtt = ddydtt_ref+Kpy*(dydt_ref-dydt)+Kiy*integral_of_y_error;
ddphiodtt = ddphidtt_ref+Kvphi*(dphidt_ref-dphidt)+Kpphi*(phi_ref-phi);

X = ddxodtt+a2*dphidt*dydt;
Y = ddyodtt-a2*dphidt*dxdt; 
PHI = ddphiodtt;

u1 = sin(phi)/(6*b1)*X+cos(phi)/(6*b1)*Y+1/(3*b2)*PHI;
u2 = -beta1/(12*b1)*X+beta3/(12*b1)*Y+1/(3*b2)*PHI;
u3 = -beta2/(12*b1)*X+beta4/(12*b1)*Y+1/(3*b2)*PHI;

y = [u1, u2, u3];
